simulink model "Studienarbeit"  (Simulink 7.1)
settings: Solver=ode45  StartTime=0.0  StopTime=10.0  RelTol=1e-3
settings Model: Creator=Castor  LastModifiedBy=Castor

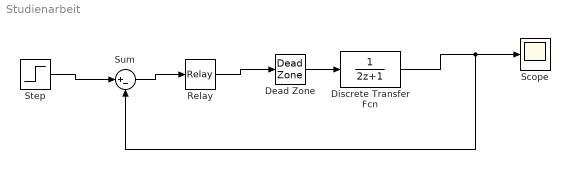
== system Studienarbeit ==
  Dead Zone : DeadZone  LowerValue=0  UpperValue=2  SaturateOnIntegerOverflow=on
  Discrete Transfer Fcn : DiscreteTransferFcn  Denominator=[2 1]
  Relay : Relay  OutDataType=sfix(16)  OutScaling=2^0
  Scope : Scope
  Step : Step  Before=-1  After=3  SampleTime=2
  Sum : Sum  Inputs=|+-  OutDataType=sfix(16)  OutScaling=2^0
  wires:
  Relay/1 -> Dead Zone/1
  Sum/1 -> Relay/1
  Step/1 -> Sum/1
  Dead Zone/1 -> Discrete Transfer Fcn/1
  Discrete Transfer Fcn/1 -> Scope/1, Sum/2
